simulink model "d10exp2_2012b"  (Simulink 8.0)
settings: Solver=ode45  SolverMode=SingleTasking  StartTime=0.0  StopTime=inf  RelTol=1e-3
libraries: powerlib x8, simulink x1
settings Model: Creator=DELL  LastModifiedBy=DELL  CovMetricSettings=dwe  CovHtmlReporting=off  covSaveCumulativeToWorkspaceVar=off  CovSaveSingleToWorkspaceVar=off  CovExternalEMLEnable=on
settings DataIOCC: LimitDataPoints=off  SaveFormat=StructureWithTime  ReturnWorkspaceOutputs=on
settings OptimizationCC: ExpressionDepthLimit=128
settings DebuggingCC: UnderspecifiedInitializationDetection=Simplified  MergeDetectMultiDrivingBlocksExec=error  SolverPrmCheckMsg=none  FrameProcessingCompatibilityMsg=error  StateNameClashWarn=none  SFUnexpectedBacktrackingDiag=error  SFNoUnconditionalDefaultTransitionDiag=error
settings HardwareCC: ProdBitPerPointer=64  ProdLargestAtomicFloat=Float  ProdIntDivRoundTo=Zero  ProdEndianess=LittleEndian  ProdHWDeviceType=Specified
settings ModelReferenceCC: PropagateSignalLabelsOutOfModel=on
settings SFSimCC: SimUseLocalCustomCode=on
settings RTWCC: RTWUseLocalCustomCode=on
settings CodeAppCC: CustomSymbolStrType=$N$R$M_T
settings GRTTargetCC: CodeReplacementLibrary=C99 (ISO)  GeneratePreprocessorConditionals=Use local settings

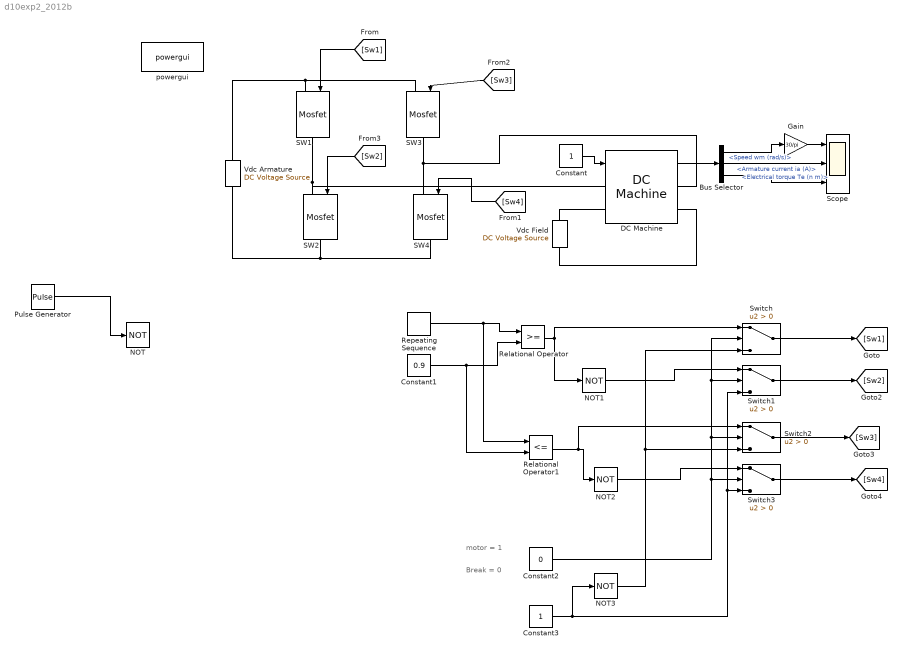
== system d10exp2_2012b ==
  note: Break = 0
  note: motor = 1
  Bus Selector : BusSelector  OutputSignals=Speed wm (rad/s),Armature current ia (A),Electrical torque Te (n m)
  Constant : Constant
  Constant1 : Constant  Value=0.9
  Constant2 : Constant  Value=0
  Constant3 : Constant
  DC Machine : powerlib/Machines/DC Machine  PresetModel=01: 5HP 240V 1750RPM Field:300V  MechanicalLoad=Torque TL  FieldType=Wound  ShowDetailedParameters=on  MeasurementBus=off  RLa=[2.581 0.028]  RLf=[281.3 156]  Laf=0.9483  MachineConstant=Torque constant (N.m/A)  Ke=1.8  Kt=1.8  J=0.02215  Bm=0.002953  Tf=0.5161  w0=1  Ifinit=1  TsPowergui=0  TsBlock=-1
  Gain : Gain  Gain=30/pi
  NOT{,1..3} (4 alike) : Logic  Operator=NOT  IconShape=distinctive  AllPortsSameDT=off  OutDataTypeStr=boolean
  Pulse Generator : DiscretePulseGenerator  PulseType=Time based  Period=1/1000  PulseWidth=25
  Relational Operator : RelationalOperator  OutDataTypeStr=boolean
  Relational Operator1 : RelationalOperator  Operator=<=  OutDataTypeStr=boolean
  Repeating Sequence : simulink/Sources/Repeating Sequence  rep_seq_t=[0 0.5 1]/1000  rep_seq_y=[0 1 0]
  SW{1..4} (4 alike) : powerlib/Power Electronics/Mosfet  Ron=0.1  Lon=0  Rd=0.01  Vfd=0  IC=0  Rs=1e5  Cs=inf  Measurements=off
  Scope : Scope  NumInputPorts=3
      settings: TimeRange=auto  MaxDataPoints=5000  SaveToWorkspace=off  SaveName=ScopeData  YMin=-22.06182~0.37479~0.38017  YMax=-2.06182~0.57479~0.58017  SampleTime=-1
  Switch{,1..3} (4 alike) : Switch  Criteria=u2 > Threshold
  Vdc Armature : powerlib/Electrical Sources/DC Voltage Source  Amplitude=240  Measurements=None
  Vdc Field : powerlib/Electrical Sources/DC Voltage Source  Amplitude=300  Measurements=None
  powergui : powerlib/powergui  Priority=1  SimulationMode=Discrete  SampleTime=50e-6  frequency=60  Iterations=50  frequencyindice=0  Pbase=100e6  ErrMax=1e-4  UnitsV=kV  UnitsW=MW  buscounter=0  FunctionMessages=off  echomessages=off  EnableUseOfTLC=off  CurrentSourceSwitches=off  DisableSnubberDevices=off  DisableRonSwitches=off  DisableVfSwitches=off  DisplayEquations=off  AutomaticDiscreteSolvers=off  SolverType=Tustin/Backward Euler (TBE)  Interpol=off  ExternalGateDelay=off  methode=off  Ts=100  x0status=blocks  SPID=on  SwTol=0  HookPort=off  NonlinearTolerance=1e-4  nMaxIteration=100  ContinueOnMaxIteration=off  RestoreLinks=warning  ResistiveCurrentMeasurement=off  Frange=[0:2:500]  Ylog=off  Xlog=on  ShowGrid=off  save=off  variable=ZData  structure=0  ZoomFFT=off  StartTime=0.0  cycles=1  DisplayStyle=1  fundamental=60  FreqAxis=off  MaxFrequency=1000  frequencyindicesteady=1  RmsSteady=1  display=off
  wires:
  DC Machine/1 -> Bus Selector/1
  Bus Selector/2 -> Scope/2  "<Armature current ia (A)>"
  Bus Selector/1 -> Gain/1  "<Speed wm (rad/s)>"
  Bus Selector/3 -> Scope/3  "<Electrical torque Te (n m)>"
  Gain/1 -> Scope/1
  Constant/1 -> DC Machine/1
  Pulse Generator/1 -> NOT/1
  [Sw1] -> SW1/1
  [Sw4] -> SW4/1
  [Sw3] -> SW3/1
  [Sw2] -> SW2/1
  Repeating Sequence/1 -> Relational Operator1/1, Relational Operator/1
  Constant1/1 -> Relational Operator1/2, Relational Operator/2
  Relational Operator/1 -> Switch/1, NOT1/1
  Relational Operator1/1 -> Switch2/1, NOT2/1
  Switch/1 -> [Sw1]
  Switch1/1 -> [Sw2]
  Switch2/1 -> [Sw3]
  Switch3/1 -> [Sw4]
  NOT1/1 -> Switch1/1
  NOT2/1 -> Switch3/1
  Constant2/1 -> Switch3/2, Switch2/2, Switch1/2, Switch/2
  Constant3/1 -> NOT3/1, Switch1/3, Switch3/3
  NOT3/1 -> Switch2/3, Switch/3
  connections:
  Vdc Field/RConn1 -- DC Machine/LConn2
  Vdc Field/LConn1 -- DC Machine/RConn2
  Vdc Armature/RConn1 -- SW3/LConn1 -- SW1/LConn1
  SW1/RConn1 -- DC Machine/LConn1 -- SW2/LConn1
  SW2/RConn1 -- Vdc Armature/LConn1 -- SW4/RConn1
  SW3/RConn1 -- DC Machine/RConn1 -- SW4/LConn1
